simulink model "lungModelsHarness"  (R2019b)
settings: Solver=VariableStepAuto  StartTime=0.0  StopTime=30  RelTol=1e-3  AbsTol=1e-3
PreLoadFcn:
  | load moistAirProperties
  | 
  | p_env = 0.101325; % MPa
  | T_env = 20; % degC
  | RH_env = 0.1;
  | y_N2_env = 0.8;
  | T_body = 37; % degC
  | 
  | comp_flow_max = 7; % l/min
  | sieve_efficiency = 0.98;
  | t_switch = 30; % s
  | open_fraction = 0.1;
  | 
  | L_tube = 1; % m
  | D_tube = 0.008; % m
  | L_trachea = 0.15; % m
  | D_trachea = 0.01; % m
  | 
  | FRC = 2; % L
  | E_respiratory = 10; % cmH2O/L
  | R_respiratory = 2; % cmH2O/(L/s)
  | 
  | % Conversion factors
  | cmH2O_to_Pa = 98.0665;
  | L_to_m3 = 1e-3;
libraries: fl_lib x22, nesl_utility x12, VentilatorLibrary x4, simulink x2
CloseFcn:
  | try,close(h1_ssc_oxygen_concentrator),end
  | clear h1_ssc_oxygen_concentrator
  | try,close(h2_ssc_oxygen_concentrator),end
  | clear h2_ssc_oxygen_concentrator
  | 
  | clear simlog_ssc_oxygen_concentrator tout
  | 
  | clear N2 O2 p_env T_env RH_env y_N2_env T_body
  | clear comp_flow_max sieve_efficiency t_switch open_fraction
  | clear L_tube D_tube L_trachea D_trachea FRC E_respiratory R_respiratory
  | clear cmH2O_to_Pa L_to_m3
Description:
  | Oxygen Concentrator
settings Model: Creator=MathWorks  LastModifiedBy=agonzale
settings SolverCC: AutoScaleAbsTol=off
settings DataIOCC: ReturnWorkspaceOutputs=off
settings DebuggingCC: PregeneratedLibrarySubsystemCodeDiagnostic=none  ArithmeticOperatorsInVariantConditions=warning
settings SFSimCC: SimUseLocalCustomCode=off  CustomCodeUndefinedFunction=UseInterfaceOnly
settings RTWCC: RTWUseLocalCustomCode=off
settings SimscapeCC: SimscapeLogType=all  SimscapeLogSimulationStatistics=on  SimscapeLogToSDI=on  SimscapeLogName=simlog_ssc_oxygen_concentrator  SimscapeLogDataHistory=25000

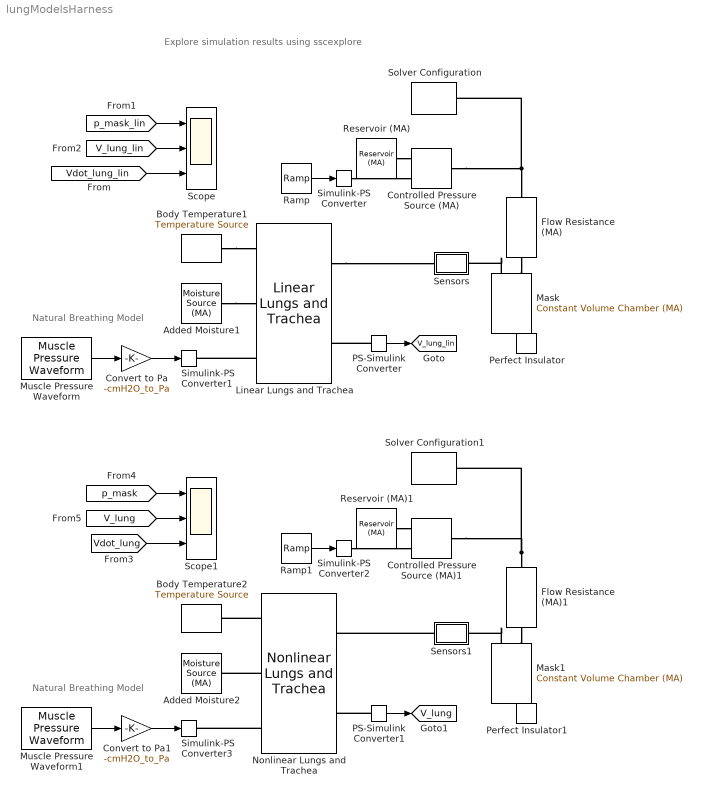
== system lungModelsHarness ==
  note: Explore simulation results using sscexplore
  note: Natural Breathing Model
  note: Natural Breathing Model
  Added Moisture1 : fl_lib/Moist Air/Sources/Moisture & Trace Gas Sources/Moisture Source (MA)  moisture_source_spec=foundation.enum.moisture_source_spec.vapor  moisture_mass_flow=0.04 g/s  temperature_spec=foundation.enum.temperature_spec.specified  moisture_temperature=35 degC
      settings: SourceProductName=Simscape  SourceProductBaseCode=SS  InternalSimscapePortConfiguration="{\"Bottom\":[],\"Left\":[{\"id\":\"S\",\"label\":\"S\",\"type\":\"foundation.moist_air.moist_air_source\"}],\"Right\":[],\"Top\":[]}"
  Added Moisture2 : fl_lib/Moist Air/Sources/Moisture & Trace Gas Sources/Moisture Source (MA)  moisture_source_spec=foundation.enum.moisture_source_spec.vapor  moisture_mass_flow=0.04 g/s  temperature_spec=foundation.enum.temperature_spec.specified  moisture_temperature=35 degC
      settings: SourceProductName=Simscape  SourceProductBaseCode=SS  InternalSimscapePortConfiguration="{\"Bottom\":[],\"Left\":[{\"id\":\"S\",\"label\":\"S\",\"type\":\"foundation.moist_air.moist_air_source\"}],\"Right\":[],\"Top\":[]}"
  Body Temperature1 : fl_lib/Thermal/Thermal Sources/Temperature Source  temperature=35 degC
      settings: SourceProductName=Simscape
  Body Temperature2 : fl_lib/Thermal/Thermal Sources/Temperature Source  temperature=35 degC
      settings: SourceProductName=Simscape
  Controlled Pressure Source (MA) : fl_lib/Moist Air/Sources/Controlled Pressure Source (MA)  power_spec=foundation.enum.power_spec.none  area_A=0.01 m^2  area_B=0.01 m^2
      settings: SourceProductName=Simscape  SourceProductBaseCode=SS  InternalSimscapePortConfiguration="{\"Bottom\":[],\"Left\":[{\"id\":\"A\",\"label\":\"A\",\"type\":\"foundation.moist_air.moist_air\"},{\"id\":\"P\",\"label\":\"P\",\"type\":\"input\"}],\"Right\":[{\"id\":\"B\",\"label\":\"B\",\"type\":\"foundation.moist_air.moist_air\"}],\"Top\":[]}"
  Controlled Pressure Source (MA)1 : fl_lib/Moist Air/Sources/Controlled Pressure Source (MA)  power_spec=foundation.enum.power_spec.none  area_A=0.01 m^2  area_B=0.01 m^2
      settings: SourceProductName=Simscape  SourceProductBaseCode=SS  InternalSimscapePortConfiguration="{\"Bottom\":[],\"Left\":[{\"id\":\"A\",\"label\":\"A\",\"type\":\"foundation.moist_air.moist_air\"},{\"id\":\"P\",\"label\":\"P\",\"type\":\"input\"}],\"Right\":[{\"id\":\"B\",\"label\":\"B\",\"type\":\"foundation.moist_air.moist_air\"}],\"Top\":[]}"
  Convert to Pa : Gain  Gain=-cmH2O_to_Pa
  Convert to Pa1 : Gain  Gain=-cmH2O_to_Pa
  Flow Resistance (MA) : fl_lib/Moist Air/Elements/Flow Resistance (MA)  delta_p_nominal=20e-3 bar  mdot_nominal=1e-3 kg/s  rho_nominal=0 kg/m^3  area=pi*D_tube^2/4 m^2  laminar_fraction=1e-3
      settings: SourceProductName=Simscape  SourceProductBaseCode=SS
  Flow Resistance (MA)1 : fl_lib/Moist Air/Elements/Flow Resistance (MA)  delta_p_nominal=20e-3 bar  mdot_nominal=1e-3 kg/s  rho_nominal=0 kg/m^3  area=pi*D_tube^2/4 m^2  laminar_fraction=1e-3
      settings: SourceProductName=Simscape  SourceProductBaseCode=SS
  Linear Lungs and Trachea : VentilatorLibrary/Linear Lungs and Trachea  FRC=2  E_respiratory=10  R_respiratory=2  vol_init=2.5  T_init=35  D_trachea=0.0150  L_trachea=0.15  A_lung_heat=0.3  h_lung=100
  Mask : fl_lib/Moist Air/Elements/Constant Volume Chamber (MA)  volume=2e-4 m^3  num_ports=foundation.enum.num_ports.two  area_A=0.01 m^2  area_B=pi*0.01^2/4 m^2  area_C=pi*D_tube^2/4 m^2  area_D=0.01 m^2  RH_ws=1  time_constant=1e-3 s  moisture_trace_gas_source=foundation.enum.moisture_trace_gas_source.none  moisture_source_spec=foundation.enum.moisture_source_spec.vapor  moisture_mass_flow=0 kg/s  moisture_temperature_spec=foundation.enum.temperature_spec.atmospheric  moisture_temperature=293.15 K  trace_gas_mass_flow=0 kg/s  trace_gas_temperature_spec=foundation.enum.temperature_spec.atmospheric  trace_gas_temperature=293.15 K  p_I_specify=off  p_I_priority=High  p_I=0.101325 MPa  p_I_nominal_specify=off  p_I_nominal_unit=MPa  p_I_nominal_value=1  T_I_specify=on  T_I_priority=High  T_I=25 degC  T_I_nominal_specify=off  T_I_nominal_unit=K  T_I_nominal_value=1  RH_I_specify=on  RH_I_priority=High  RH_I=0.1  RH_I_nominal_specify=off  RH_I_nominal_unit=1  RH_I_nominal_value=1  x_w_I_specify=off  x_w_I_priority=None  x_w_I=0  x_w_I_nominal_specify=off  x_w_I_nominal_unit=1  x_w_I_nominal_value=1  y_w_I_specify=off  y_w_I_priority=None  y_w_I=0  y_w_I_nominal_specify=off  y_w_I_nominal_unit=1  y_w_I_nominal_value=1  HR_I_specify=off  HR_I_priority=None  HR_I=0  HR_I_nominal_specify=off  HR_I_nominal_unit=1  HR_I_nominal_value=1  x_g_I_specify=on  x_g_I_priority=None  x_g_I=0  x_g_I_nominal_specify=off  x_g_I_nominal_unit=1  x_g_I_nominal_value=1  y_g_I_specify=on  y_g_I_priority=High  y_g_I=0.7  y_g_I_nominal_specify=off  y_g_I_nominal_unit=1  y_g_I_nominal_value=1
      settings: SourceProductName=Simscape  SourceProductBaseCode=SS  InternalSimscapePortConfiguration="{\"Bottom\":[],\"Left\":[{\"id\":\"A\",\"label\":\"A\",\"type\":\"foundation.moist_air.moist_air\"},{\"id\":\"B\",\"label\":\"B\",\"type\":\"foundation.moist_air.moist_air\"}],\"Right\":[{\"id\":\"W\",\"label\":\"W\",\"type\":\"output\"},{\"id\":\"F\",\"label\":\"F\",\"type\":\"output\"},{\"id\":\"H\",\"label\":\"H\",\"type\":\"foundation.thermal.thermal\"}],\"Top\":[]}"
  Mask1 : fl_lib/Moist Air/Elements/Constant Volume Chamber (MA)  volume=2e-4 m^3  num_ports=foundation.enum.num_ports.two  area_A=0.01 m^2  area_B=pi*0.01^2/4 m^2  area_C=pi*D_tube^2/4 m^2  area_D=0.01 m^2  RH_ws=1  time_constant=1e-3 s  moisture_trace_gas_source=foundation.enum.moisture_trace_gas_source.none  moisture_source_spec=foundation.enum.moisture_source_spec.vapor  moisture_mass_flow=0 kg/s  moisture_temperature_spec=foundation.enum.temperature_spec.atmospheric  moisture_temperature=293.15 K  trace_gas_mass_flow=0 kg/s  trace_gas_temperature_spec=foundation.enum.temperature_spec.atmospheric  trace_gas_temperature=293.15 K  p_I_specify=off  p_I_priority=High  p_I=0.101325 MPa  p_I_nominal_specify=off  p_I_nominal_unit=MPa  p_I_nominal_value=1  T_I_specify=on  T_I_priority=High  T_I=25 degC  T_I_nominal_specify=off  T_I_nominal_unit=K  T_I_nominal_value=1  RH_I_specify=on  RH_I_priority=High  RH_I=0.1  RH_I_nominal_specify=off  RH_I_nominal_unit=1  RH_I_nominal_value=1  x_w_I_specify=off  x_w_I_priority=None  x_w_I=0  x_w_I_nominal_specify=off  x_w_I_nominal_unit=1  x_w_I_nominal_value=1  y_w_I_specify=off  y_w_I_priority=None  y_w_I=0  y_w_I_nominal_specify=off  y_w_I_nominal_unit=1  y_w_I_nominal_value=1  HR_I_specify=off  HR_I_priority=None  HR_I=0  HR_I_nominal_specify=off  HR_I_nominal_unit=1  HR_I_nominal_value=1  x_g_I_specify=on  x_g_I_priority=None  x_g_I=0  x_g_I_nominal_specify=off  x_g_I_nominal_unit=1  x_g_I_nominal_value=1  y_g_I_specify=on  y_g_I_priority=High  y_g_I=0.7  y_g_I_nominal_specify=off  y_g_I_nominal_unit=1  y_g_I_nominal_value=1
      settings: SourceProductName=Simscape  SourceProductBaseCode=SS  InternalSimscapePortConfiguration="{\"Bottom\":[],\"Left\":[{\"id\":\"A\",\"label\":\"A\",\"type\":\"foundation.moist_air.moist_air\"},{\"id\":\"B\",\"label\":\"B\",\"type\":\"foundation.moist_air.moist_air\"}],\"Right\":[{\"id\":\"W\",\"label\":\"W\",\"type\":\"output\"},{\"id\":\"F\",\"label\":\"F\",\"type\":\"output\"},{\"id\":\"H\",\"label\":\"H\",\"type\":\"foundation.thermal.thermal\"}],\"Top\":[]}"
  Muscle Pressure Waveform : VentilatorLibrary/Muscle Pressure Waveform  p_muscle_mag=5  t_inhale=0.3  t_exhale=0.7  period=3
  Muscle Pressure Waveform1 : VentilatorLibrary/Muscle Pressure Waveform  p_muscle_mag=5  t_inhale=0.3  t_exhale=0.7  period=3
  Nonlinear Lungs and Trachea : VentilatorLibrary/Nonlinear Lungs and Trachea  Vmax=5  FRC=2  E_respiratory=10  R_respiratory=2  vol_init=2.5  T_init=35  D_trachea=0.0150  L_trachea=0.15  A_lung_heat=0.3  h_lung=100
  PS-Simulink Converter : nesl_utility/PS-Simulink Converter  PhysicalDomain=network_engine_domain  SubClassName=ps_output  LeftPortType=input  RightPortType=output  PseudoPeriodic=off  Frequencies=[]  Unit=l  AffineConversion=off
  PS-Simulink Converter1 : nesl_utility/PS-Simulink Converter  PhysicalDomain=network_engine_domain  SubClassName=ps_output  LeftPortType=input  RightPortType=output  PseudoPeriodic=off  Frequencies=[]  Unit=l  AffineConversion=off
  Perfect Insulator : fl_lib/Thermal/Thermal Elements/Perfect Insulator  T_specify=off  T_priority=None  T=0 K  T_nominal_specify=off  T_nominal_unit=K  T_nominal_value=1
      settings: SourceProductName=Simscape
  Perfect Insulator1 : fl_lib/Thermal/Thermal Elements/Perfect Insulator  T_specify=off  T_priority=None  T=0 K  T_nominal_specify=off  T_nominal_unit=K  T_nominal_value=1
      settings: SourceProductName=Simscape
  Ramp : simulink/Sources/Ramp  slope=1000e-3/15  start=15  InitialOutput=0
  Ramp1 : simulink/Sources/Ramp  slope=1000e-3/15  start=15  InitialOutput=0
  Reservoir (MA) : fl_lib/Moist Air/Elements/Reservoir (MA)  pressure_spec=foundation.enum.pressure_spec.atmospheric  reservoir_pressure=0.101325 MPa  temperature_spec=foundation.enum.temperature_spec.atmospheric  reservoir_temperature=293.15 K  moisture_spec=foundation.enum.moisture_spec.relative_humidity  reservoir_RH=0.1  reservoir_x_w=0.01  reservoir_y_w=0.01  reservoir_HR=0.01  trace_gas_spec=foundation.enum.trace_gas_spec.mole_fraction  reservoir_x_g=0.001  reservoir_y_g=0.7  RH_ws=1  area_A=0.01 m^2
      settings: SourceProductName=Simscape  SourceProductBaseCode=SS
  Reservoir (MA)1 : fl_lib/Moist Air/Elements/Reservoir (MA)  pressure_spec=foundation.enum.pressure_spec.atmospheric  reservoir_pressure=0.101325 MPa  temperature_spec=foundation.enum.temperature_spec.atmospheric  reservoir_temperature=293.15 K  moisture_spec=foundation.enum.moisture_spec.relative_humidity  reservoir_RH=0.1  reservoir_x_w=0.01  reservoir_y_w=0.01  reservoir_HR=0.01  trace_gas_spec=foundation.enum.trace_gas_spec.mole_fraction  reservoir_x_g=0.001  reservoir_y_g=0.7  RH_ws=1  area_A=0.01 m^2
      settings: SourceProductName=Simscape  SourceProductBaseCode=SS
  Scope : Scope  NumInputPorts=3
  Scope1 : Scope  NumInputPorts=3
  Sensors : Subsystem
  Sensors1 : Subsystem
  Simulink-PS Converter : nesl_utility/Simulink-PS Converter  PhysicalDomain=network_engine_domain  SubClassName=ps_input  LeftPortType=input  RightPortType=output  PseudoPeriodic=off  Frequencies=[]  NoiseDistribution=none  NoiseParameters=[]  Unit=bar  AffineConversion=off  FilteringAndDerivatives=provide  SimscapeFilterOrder=1  InputFilterTimeConstant=0.001  UdotUserProvided=0
  Simulink-PS Converter1 : nesl_utility/Simulink-PS Converter  PhysicalDomain=network_engine_domain  SubClassName=ps_input  LeftPortType=input  RightPortType=output  PseudoPeriodic=off  Frequencies=[]  NoiseDistribution=none  NoiseParameters=[]  Unit=Pa  AffineConversion=off  FilteringAndDerivatives=provide  SimscapeFilterOrder=1  InputFilterTimeConstant=0.001  UdotUserProvided=0
  Simulink-PS Converter2 : nesl_utility/Simulink-PS Converter  PhysicalDomain=network_engine_domain  SubClassName=ps_input  LeftPortType=input  RightPortType=output  PseudoPeriodic=off  Frequencies=[]  NoiseDistribution=none  NoiseParameters=[]  Unit=bar  AffineConversion=off  FilteringAndDerivatives=provide  SimscapeFilterOrder=1  InputFilterTimeConstant=0.001  UdotUserProvided=0
  Simulink-PS Converter3 : nesl_utility/Simulink-PS Converter  PhysicalDomain=network_engine_domain  SubClassName=ps_input  LeftPortType=input  RightPortType=output  PseudoPeriodic=off  Frequencies=[]  NoiseDistribution=none  NoiseParameters=[]  Unit=Pa  AffineConversion=off  FilteringAndDerivatives=provide  SimscapeFilterOrder=1  InputFilterTimeConstant=0.001  UdotUserProvided=0
  Solver Configuration : nesl_utility/Solver Configuration  PhysicalDomain=network_engine_domain  SubClassName=solver  LeftPortType=input  RightPortType=generic  Tones=[]  Harmonics=[]  SimulateNoise=off  Profile=off  UseLocalSampling=off  EnableSwitchedLinearOptims=on  FrequencyDomain=off  UseCCode=off  RelTol=0.001  AbsTol=1e-06  MinStep=1e-09  ToWorkspace=off  RevertToSquareIcSolve=off  NumHomotopyIterations=100  PhasorMode=off  PhasorModeNumHarmonics=1  DoDC=off  ResidualTolerance=1e-09  UseLocalSolver=off  LocalSolverChoice=NE_BACKWARD_EULER_ADVANCER  LocalSolverSampleTime=0.001  DoFixedCost=off  MaxNonlinIter=3  MaxModeIter=2  LinearAlgebra=auto  EquationFormulation=NE_TIME_EF  DelaysMemoryBudget=1024  AutomaticFiltering=on  FilteringTimeConstant=0.001  PartitionStorageMethod=AS_NEEDED  PartitionMemoryBudget=1024  PartitionMethod=ROBUST
  Solver Configuration1 : nesl_utility/Solver Configuration  PhysicalDomain=network_engine_domain  SubClassName=solver  LeftPortType=input  RightPortType=generic  Tones=[]  Harmonics=[]  SimulateNoise=off  Profile=off  UseLocalSampling=off  EnableSwitchedLinearOptims=on  FrequencyDomain=off  UseCCode=off  RelTol=0.001  AbsTol=1e-06  MinStep=1e-09  ToWorkspace=off  RevertToSquareIcSolve=off  NumHomotopyIterations=100  PhasorMode=off  PhasorModeNumHarmonics=1  DoDC=off  ResidualTolerance=1e-09  UseLocalSolver=off  LocalSolverChoice=NE_BACKWARD_EULER_ADVANCER  LocalSolverSampleTime=0.001  DoFixedCost=off  MaxNonlinIter=3  MaxModeIter=2  LinearAlgebra=auto  EquationFormulation=NE_TIME_EF  DelaysMemoryBudget=1024  AutomaticFiltering=on  FilteringTimeConstant=0.001  PartitionStorageMethod=AS_NEEDED  PartitionMemoryBudget=1024  PartitionMethod=ROBUST
  tag scope: V_lung=global, V_lung_lin=global
  wires:
  Ramp/1 -> Simulink-PS Converter/1
  [p_mask_lin] -> Scope/1
  [V_lung_lin] -> Scope/2
  [Vdot_lung_lin] -> Scope/3
  PS-Simulink Converter/1 -> [V_lung_lin]
  Muscle Pressure Waveform/1 -> Convert to Pa/1
  Convert to Pa/1 -> Simulink-PS Converter1/1
  Convert to Pa1/1 -> Simulink-PS Converter3/1
  Ramp1/1 -> Simulink-PS Converter2/1
  [p_mask] -> Scope1/1
  [V_lung] -> Scope1/2
  Muscle Pressure Waveform1/1 -> Convert to Pa1/1
  PS-Simulink Converter1/1 -> [V_lung]
  [Vdot_lung] -> Scope1/3
  connections:
  Mask/RConn3 -- Perfect Insulator/LConn1
  Mask/LConn1 -- Sensors/LConn1
  Controlled Pressure Source (MA)/RConn1 -- Solver Configuration/RConn1 -- Flow Resistance (MA)/LConn1
  Reservoir (MA)/LConn1 -- Controlled Pressure Source (MA)/LConn1
  Simulink-PS Converter/RConn1 -- Controlled Pressure Source (MA)/LConn2
  Flow Resistance (MA)/RConn1 -- Mask/LConn2
  Linear Lungs and Trachea/LConn3 -- Simulink-PS Converter1/RConn1
  Body Temperature1/LConn1 -- Linear Lungs and Trachea/LConn1
  Added Moisture1/LConn1 -- Linear Lungs and Trachea/LConn2
  Linear Lungs and Trachea/RConn1 -- Sensors/RConn1
  PS-Simulink Converter/LConn1 -- Linear Lungs and Trachea/RConn2
  Flow Resistance (MA)1/LConn1 -- Solver Configuration1/RConn1 -- Controlled Pressure Source (MA)1/RConn1
  Flow Resistance (MA)1/RConn1 -- Mask1/LConn2
  Reservoir (MA)1/LConn1 -- Controlled Pressure Source (MA)1/LConn1
  PS-Simulink Converter1/LConn1 -- Nonlinear Lungs and Trachea/RConn2
  Nonlinear Lungs and Trachea/LConn1 -- Body Temperature2/LConn1
  Simulink-PS Converter2/RConn1 -- Controlled Pressure Source (MA)1/LConn2
  Mask1/LConn1 -- Sensors1/LConn1
  Sensors1/RConn1 -- Nonlinear Lungs and Trachea/RConn1
  Mask1/RConn3 -- Perfect Insulator1/LConn1
  Nonlinear Lungs and Trachea/LConn2 -- Added Moisture2/LConn1
  Nonlinear Lungs and Trachea/LConn3 -- Simulink-PS Converter3/RConn1

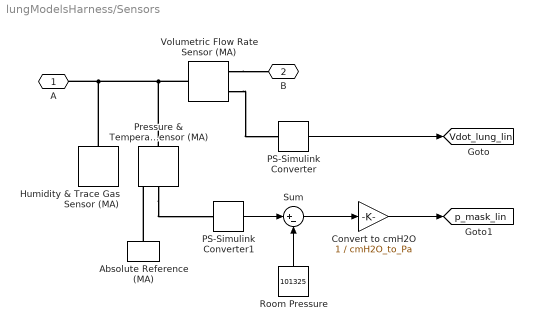
== system lungModelsHarness/Sensors ==
  Absolute Reference (MA) : fl_lib/Moist Air/Elements/Absolute Reference (MA)
      settings: SourceProductName=Simscape  SourceProductBaseCode=SS
  Convert to cmH2O : Gain  Gain=1 / cmH2O_to_Pa
  Humidity & Trace Gas Sensor (MA) : fl_lib/Moist Air/Sensors/Humidity & Trace Gas Sensor (MA)  moisture_spec=foundation.enum.moisture_spec.relative_humidity  trace_gas_spec=foundation.enum.trace_gas_spec.mass_fraction
      settings: SourceProductName=Simscape  SourceProductBaseCode=SS  InternalSimscapePortConfiguration="{\"Bottom\":[],\"Left\":[{\"id\":\"A\",\"label\":\"A\",\"type\":\"foundation.moist_air.moist_air\"}],\"Right\":[{\"id\":\"W\",\"label\":\"W\",\"type\":\"output\"},{\"id\":\"G\",\"label\":\"G\",\"type\":\"output\"}],\"Top\":[]}"
  PS-Simulink Converter : nesl_utility/PS-Simulink Converter  PhysicalDomain=network_engine_domain  SubClassName=ps_output  LeftPortType=input  RightPortType=output  PseudoPeriodic=off  Frequencies=[]  Unit=lpm  AffineConversion=off
  PS-Simulink Converter1 : nesl_utility/PS-Simulink Converter  PhysicalDomain=network_engine_domain  SubClassName=ps_output  LeftPortType=input  RightPortType=output  PseudoPeriodic=off  Frequencies=[]  Unit=Pa  AffineConversion=off
  Pressure & Temperature Sensor (MA) : fl_lib/Moist Air/Sensors/Pressure & Temperature Sensor (MA)
      settings: SourceProductName=Simscape  SourceProductBaseCode=SS  InternalSimscapePortConfiguration="{\"Bottom\":[],\"Left\":[{\"id\":\"A\",\"label\":\"A\",\"type\":\"foundation.moist_air.moist_air\"}],\"Right\":[{\"id\":\"B\",\"label\":\"B\",\"type\":\"foundation.moist_air.moist_air\"},{\"id\":\"P\",\"label\":\"P\",\"type\":\"output\"},{\"id\":\"T\",\"label\":\"T\",\"type\":\"output\"}],\"Top\":[]}"
  Room Pressure : Constant  Value=101325
  Sum : Sum  Inputs=|+-
  Volumetric Flow Rate Sensor (MA) : fl_lib/Moist Air/Sensors/Volumetric Flow Rate Sensor (MA)  volumetric_flow_conditions=foundation.enum.volumetric_flow_conditions.actual  p_std=0.101325 MPa  T_std=20 degC  RH_std=0.65
      settings: SourceProductName=Simscape  SourceProductBaseCode=SS  InternalSimscapePortConfiguration="{\"Bottom\":[],\"Left\":[{\"id\":\"A\",\"label\":\"A\",\"type\":\"foundation.moist_air.moist_air\"}],\"Right\":[{\"id\":\"B\",\"label\":\"B\",\"type\":\"foundation.moist_air.moist_air\"},{\"id\":\"V\",\"label\":\"V\",\"type\":\"output\"}],\"Top\":[]}"
  A : PMIOPort  Side=Left
  B : PMIOPort  Port=2  Side=Right
  tag scope: Vdot_lung_lin=global, p_mask_lin=global
  wires:
  PS-Simulink Converter/1 -> [Vdot_lung_lin]
  Convert to cmH2O/1 -> [p_mask_lin]
  PS-Simulink Converter1/1 -> Sum/1
  Sum/1 -> Convert to cmH2O/1
  Room Pressure/1 -> Sum/2
  connections:
  Volumetric Flow Rate Sensor (MA)/LConn1 -- Pressure & Temperature Sensor (MA)/LConn1 -- Humidity & Trace Gas Sensor (MA)/LConn1 -- A/RConn1
  Volumetric Flow Rate Sensor (MA)/RConn1 -- B/RConn1
  Volumetric Flow Rate Sensor (MA)/RConn2 -- PS-Simulink Converter/LConn1
  Absolute Reference (MA)/LConn1 -- Pressure & Temperature Sensor (MA)/RConn1
  Pressure & Temperature Sensor (MA)/RConn2 -- PS-Simulink Converter1/LConn1

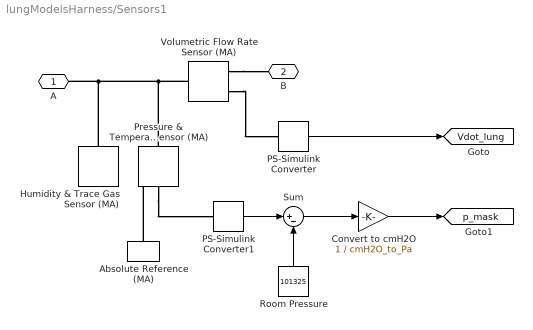
== system lungModelsHarness/Sensors1 ==
  Absolute Reference (MA) : fl_lib/Moist Air/Elements/Absolute Reference (MA)
      settings: SourceProductName=Simscape  SourceProductBaseCode=SS
  Convert to cmH2O : Gain  Gain=1 / cmH2O_to_Pa
  Humidity & Trace Gas Sensor (MA) : fl_lib/Moist Air/Sensors/Humidity & Trace Gas Sensor (MA)  moisture_spec=foundation.enum.moisture_spec.relative_humidity  trace_gas_spec=foundation.enum.trace_gas_spec.mass_fraction
      settings: SourceProductName=Simscape  SourceProductBaseCode=SS  InternalSimscapePortConfiguration="{\"Bottom\":[],\"Left\":[{\"id\":\"A\",\"label\":\"A\",\"type\":\"foundation.moist_air.moist_air\"}],\"Right\":[{\"id\":\"W\",\"label\":\"W\",\"type\":\"output\"},{\"id\":\"G\",\"label\":\"G\",\"type\":\"output\"}],\"Top\":[]}"
  PS-Simulink Converter : nesl_utility/PS-Simulink Converter  PhysicalDomain=network_engine_domain  SubClassName=ps_output  LeftPortType=input  RightPortType=output  PseudoPeriodic=off  Frequencies=[]  Unit=lpm  AffineConversion=off
  PS-Simulink Converter1 : nesl_utility/PS-Simulink Converter  PhysicalDomain=network_engine_domain  SubClassName=ps_output  LeftPortType=input  RightPortType=output  PseudoPeriodic=off  Frequencies=[]  Unit=Pa  AffineConversion=off
  Pressure & Temperature Sensor (MA) : fl_lib/Moist Air/Sensors/Pressure & Temperature Sensor (MA)
      settings: SourceProductName=Simscape  SourceProductBaseCode=SS  InternalSimscapePortConfiguration="{\"Bottom\":[],\"Left\":[{\"id\":\"A\",\"label\":\"A\",\"type\":\"foundation.moist_air.moist_air\"}],\"Right\":[{\"id\":\"B\",\"label\":\"B\",\"type\":\"foundation.moist_air.moist_air\"},{\"id\":\"P\",\"label\":\"P\",\"type\":\"output\"},{\"id\":\"T\",\"label\":\"T\",\"type\":\"output\"}],\"Top\":[]}"
  Room Pressure : Constant  Value=101325
  Sum : Sum  Inputs=|+-
  Volumetric Flow Rate Sensor (MA) : fl_lib/Moist Air/Sensors/Volumetric Flow Rate Sensor (MA)  volumetric_flow_conditions=foundation.enum.volumetric_flow_conditions.actual  p_std=0.101325 MPa  T_std=20 degC  RH_std=0.65
      settings: SourceProductName=Simscape  SourceProductBaseCode=SS  InternalSimscapePortConfiguration="{\"Bottom\":[],\"Left\":[{\"id\":\"A\",\"label\":\"A\",\"type\":\"foundation.moist_air.moist_air\"}],\"Right\":[{\"id\":\"B\",\"label\":\"B\",\"type\":\"foundation.moist_air.moist_air\"},{\"id\":\"V\",\"label\":\"V\",\"type\":\"output\"}],\"Top\":[]}"
  A : PMIOPort  Side=Left
  B : PMIOPort  Port=2  Side=Right
  tag scope: Vdot_lung=global, p_mask=global
  wires:
  PS-Simulink Converter/1 -> [Vdot_lung]
  Convert to cmH2O/1 -> [p_mask]
  PS-Simulink Converter1/1 -> Sum/1
  Sum/1 -> Convert to cmH2O/1
  Room Pressure/1 -> Sum/2
  connections:
  Volumetric Flow Rate Sensor (MA)/LConn1 -- Pressure & Temperature Sensor (MA)/LConn1 -- Humidity & Trace Gas Sensor (MA)/LConn1 -- A/RConn1
  Volumetric Flow Rate Sensor (MA)/RConn1 -- B/RConn1
  Volumetric Flow Rate Sensor (MA)/RConn2 -- PS-Simulink Converter/LConn1
  Absolute Reference (MA)/LConn1 -- Pressure & Temperature Sensor (MA)/RConn1
  Pressure & Temperature Sensor (MA)/RConn2 -- PS-Simulink Converter1/LConn1
